simulink model "forward_ideal"  (R2018a)
settings: Solver=VariableStepAuto  StartTime=0.0  StopTime=1  RelTol=1e-3
undefined symbols (not defined in the file or in its folder): DC, Duty, freq, Lm
libraries: powerlib x16, powerlib_meascontrol x2
settings Model: Creator=Emre Deniz  LastModifiedBy=Emre Deniz
settings DebuggingCC: UnconnectedInputMsg=none  UnconnectedOutputMsg=none  UnconnectedLineMsg=none

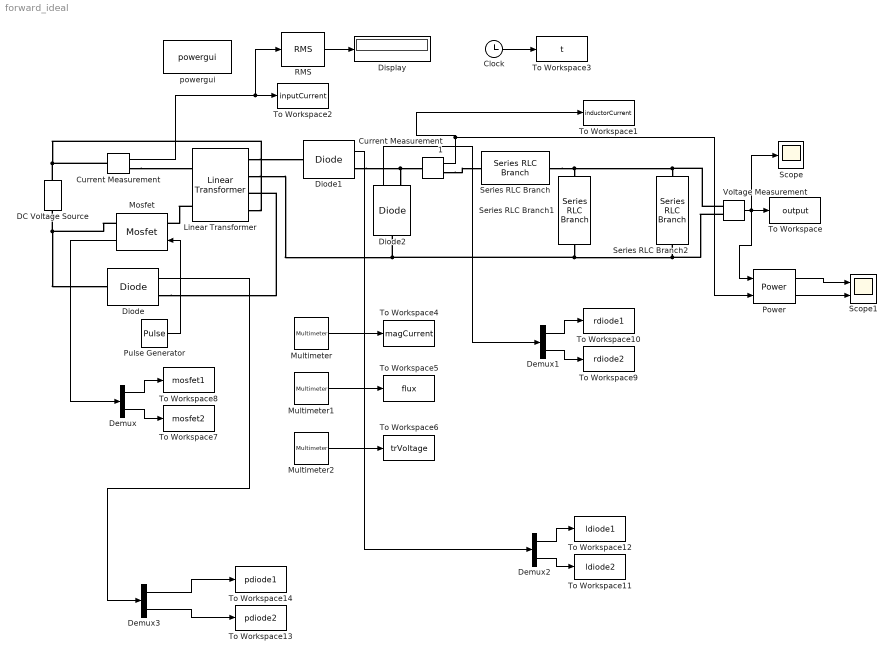
== system forward_ideal ==
  Clock : Clock
  Current Measurement : powerlib/Measurements/Current Measurement  PhasorSimulation=off  OutputType=Complex  PSBequivalent=0
  Current Measurement1 : powerlib/Measurements/Current Measurement  PhasorSimulation=off  OutputType=Complex  PSBequivalent=0
  DC Voltage Source : powerlib/Electrical Sources/DC Voltage Source  Amplitude=DC  Measurements=None
  Demux{,1..3} (4 alike) : Demux  Outputs=2
  Diode : powerlib/Power Electronics/Diode  Ron=0.001  Lon=0  Vf=V_f  IC=0  UseSnubber=0  Rs=500  Cs=250e-9  Measurements=on
  Diode1 : powerlib/Power Electronics/Diode  Ron=0.001  Lon=0  Vf=V_f  IC=0  UseSnubber=0  Rs=500  Cs=250e-9  Measurements=on
  Diode2 : powerlib/Power Electronics/Diode  Ron=0.001  Lon=0  Vf=V_f  IC=0  UseSnubber=0  Rs=500  Cs=250e-9  Measurements=on
  Display : Display
  Linear Transformer : powerlib/Elements/Linear Transformer  UNITS=SI  NominalPower=[48 25e3 ]  winding1=[ 48 0.02 0]  winding2=[ 72 0.02 0]  ThreeWindings=on  winding3=[ 48 0.02 0]  RmLm=[500e6 Lm]  Measurements=All voltages and currents  DataType=on
  Mosfet : powerlib/Power Electronics/Mosfet  Ron=0.03  Lon=0  Rd=1e-3  Vfd=0  IC=0  Rs=1e5  Cs=inf  Measurements=on
  Multimeter : powerlib/Measurements/Multimeter  PhasorSimulation=off  OutputType=Complex  sel=7  L=9  Gain=1  yselected={'Iexc: Linear Transformer'};  PSBOutputType=1  PSBequivalent=0  AxesSetting=[0,0.1,-100,100]  Display=0  SavedBlockNames=-11
  Multimeter1 : powerlib/Measurements/Multimeter  PhasorSimulation=off  OutputType=Complex  sel=9  L=9  Gain=1  yselected={'Flux: Linear Transformer'};  PSBOutputType=1  PSBequivalent=0  AxesSetting=[0,0.1,-100,100]  Display=0  SavedBlockNames=-11
  Multimeter2 : powerlib/Measurements/Multimeter  PhasorSimulation=off  OutputType=Complex  sel=[1 2 3]  L=9  Gain=[1 1 1]  yselected={'Uw1: Linear Transformer','Uw2: Linear Transformer','Uw3: Linear Transformer'};  PSBOutputType=1  PSBequivalent=0  AxesSetting=[0,0.1,-100,100]  Display=0  SavedBlockNames=-11
  Power : powerlib_meascontrol/Measurements/Power  Freq=60  Vinit=[1, 0]  Iinit=[1, 0]  Ts=0
      settings: SourceProductName=Simscape Power Systems
  Pulse Generator : DiscretePulseGenerator  PulseType=Time based  Amplitude=5  Period=1/freq  PulseWidth=Duty
  RMS : powerlib_meascontrol/Measurements/RMS  TrueRMS=on  Freq=60  RMSInit=120  Ts=0
  Scope : Scope
  Scope1 : Scope  NumInputPorts=2
  Series RLC Branch : powerlib/Elements/Series RLC Branch  LConnTagsString=__new0  RConnTagsString=__new0  BranchType=RL  Resistance=60e-3  Inductance=0.675e-3  SetiL0=off  InitialCurrent=0  Capacitance=1e-6  Setx0=off  InitialVoltage=0  Measurements=None
  Series RLC Branch1 : powerlib/Elements/Series RLC Branch  LConnTagsString=__new0  RConnTagsString=__new0  BranchType=RC  Resistance=3e-3  Inductance=1e-3  SetiL0=off  InitialCurrent=0  Capacitance=30e-6  Setx0=off  InitialVoltage=0  Measurements=None
  Series RLC Branch2 : powerlib/Elements/Series RLC Branch  LConnTagsString=__new0  RConnTagsString=__new0  BranchType=R  Resistance=15/3.2  Inductance=1e-3  SetiL0=off  InitialCurrent=0  Capacitance=1e-6  Setx0=off  InitialVoltage=0  Measurements=None
  To Workspace : ToWorkspace  VariableName=output  SampleTime=-1
  To Workspace1 : ToWorkspace  VariableName=inductorCurrent  SampleTime=-1
  To Workspace10 : ToWorkspace  VariableName=rdiode1  SampleTime=-1
  To Workspace11 : ToWorkspace  VariableName=ldiode2  SampleTime=-1
  To Workspace12 : ToWorkspace  VariableName=ldiode1  SampleTime=-1
  To Workspace13 : ToWorkspace  VariableName=pdiode2  SampleTime=-1
  To Workspace14 : ToWorkspace  VariableName=pdiode1  SampleTime=-1
  To Workspace2 : ToWorkspace  VariableName=inputCurrent  SampleTime=-1
  To Workspace3 : ToWorkspace  VariableName=t  SampleTime=-1
  To Workspace4 : ToWorkspace  VariableName=magCurrent  SampleTime=-1
  To Workspace5 : ToWorkspace  VariableName=flux  SampleTime=-1
  To Workspace6 : ToWorkspace  VariableName=trVoltage  SampleTime=-1
  To Workspace7 : ToWorkspace  VariableName=mosfet2  SampleTime=-1
  To Workspace8 : ToWorkspace  VariableName=mosfet1  SampleTime=-1
  To Workspace9 : ToWorkspace  VariableName=rdiode2  SampleTime=-1
  Voltage Measurement : powerlib/Measurements/Voltage Measurement  PhasorSimulation=off  OutputType=Complex  PSBequivalent=0
  powergui : powerlib/powergui  Priority=1  SimulationMode=Continuous  SampleTime=50e-6  frequency=60  Iterations=50  frequencyindice=0  Pbase=100e6  ErrMax=1e-4  UnitsV=kV  UnitsW=MW  buscounter=0  FunctionMessages=off  echomessages=off  EnableUseOfTLC=off  CurrentSourceSwitches=off  DisableSnubberDevices=off  DisableRonSwitches=off  DisableVfSwitches=off  DisplayEquations=off  SolverType=Tustin/Backward Euler (TBE)  Interpol=off  ExternalGateDelay=off  methode=off  Ts=100  x0status=blocks  SPID=on  SwTol=0  HookPort=off  RestoreLinks=warning  ResistiveCurrentMeasurement=off  Frange=[0:2:500]  Ylog=off  Xlog=on  ShowGrid=off  save=off  variable=ZData  structure=0  ZoomFFT=off  StartTime=0.0  cycles=1  DisplayStyle=1  fundamental=60  FreqAxis=off  MaxFrequency=1000  frequencyindicesteady=1  RmsSteady=1  display=off
  wires:
  Pulse Generator/1 -> Mosfet/1
  Voltage Measurement/1 -> Power/1, Scope/1, To Workspace/1
  Current Measurement1/1 -> Power/2, To Workspace1/1
  Current Measurement/1 -> RMS/1, To Workspace2/1
  Clock/1 -> To Workspace3/1
  Multimeter/1 -> To Workspace4/1
  Multimeter1/1 -> To Workspace5/1
  Multimeter2/1 -> To Workspace6/1
  RMS/1 -> Display/1
  Mosfet/1 -> Demux/1
  Demux/1 -> To Workspace8/1
  Demux/2 -> To Workspace7/1
  Demux1/1 -> To Workspace10/1
  Demux1/2 -> To Workspace9/1
  Diode2/1 -> Demux1/1
  Demux2/1 -> To Workspace12/1
  Demux2/2 -> To Workspace11/1
  Diode1/1 -> Demux2/1
  Demux3/1 -> To Workspace14/1
  Demux3/2 -> To Workspace13/1
  Diode/1 -> Demux3/1
  Power/1 -> Scope1/1
  Power/2 -> Scope1/2
  connections:
  DC Voltage Source/RConn1 -- Linear Transformer/RConn4 -- Current Measurement/LConn1
  Linear Transformer/LConn2 -- Mosfet/LConn1
  Mosfet/RConn1 -- Diode/LConn1 -- DC Voltage Source/LConn1
  Linear Transformer/RConn1 -- Diode1/LConn1
  Diode1/RConn1 -- Current Measurement1/LConn1 -- Diode2/RConn1
  Series RLC Branch1/RConn1 -- Linear Transformer/RConn2 -- Diode2/LConn1 -- Voltage Measurement/LConn2 -- Series RLC Branch2/RConn1
  Series RLC Branch/RConn1 -- Voltage Measurement/LConn1 -- Series RLC Branch2/LConn1 -- Series RLC Branch1/LConn1
  Current Measurement/RConn1 -- Linear Transformer/LConn1
  Current Measurement1/RConn1 -- Series RLC Branch/LConn1
  Diode/RConn1 -- Linear Transformer/RConn3
